simulink model "ADU_Integration_R2014a_simulation"  (R2014a)
settings: Solver=FixedStepDiscrete  StartTime=285  StopTime=300  FixedStep=0.01  RelTol=1e-3
PostLoadFcn:
  | , if any(exist('dsrtsu_mdlpostloadfcn', 'file') == [2, 3, 6]), try dsrtsu_mdlpostloadfcn('Execute', bdroot); catch fprintf('Error in PostLoadFcn (dsrtsu_mdlpostloadfcn) for model "%s":\n %s\n', bdroot, lasterr); end, end,
InitFcn:
  | load 'data/chi2_dat';
  | load 'data/Line_struct';
  | load 'data/innerLNM_1';
  | load 'data/middleLNM_2';
  | load 'data/outerLNM_1';
  | load 'data/landmarks_patac_schimmel_ccw';
  | load 'data/patac_navi_array';
  | load 'data/sensor';
  | load 'data/map_struct';
  | addpath map_src
  | Integration_Parameter;
  | load 'TestData_001';
values from neighbouring files (symbols this model uses):
  TestData_001 =     [TestData_001.mat]
undefined symbols (not defined in the file or in its folder): chi2_dat, innerLNM_1, landmarks_patac_schimmel_ccw, middleLNM_2, outerLNM_1, patac_navi_array
libraries: simulink x36, rtican x1
(part 12 of 22)

== matlab function ADU_Integration_R2014a_simulation/Path_Plan/CordTransfer ==
  data: Info_MeGCd input; Info_MePGCd output size=1,6; RoadInfoPGCd output size=2,4; Info_FdGCd input; Info_FoGCd input; Info_LdGCd input; Info_LoGCd input; CurOpGCd input; LongDisLimitGCd input; RoadInfoGCd input; Info_FdPGCd output size=1,6; Info_FoPGCd output size=1,6; Info_LdPGCd output size=1,6; Info_LoPGCd output size=1,6; LongDisLimitPGCd output; CurOpPGCd output; PGCdInfo output size=1,3
function [Info_MePGCd,RoadInfoPGCd,Info_FdPGCd,Info_FoPGCd,Info_LdPGCd,Info_LoPGCd,LongDisLimitPGCd,CurOpPGCd,PGCdInfo] = CordTransfer(Info_MeGCd,Info_FdGCd,Info_FoGCd,Info_LdGCd,Info_LoGCd,CurOpGCd,LongDisLimitGCd,RoadInfoGCd)
%#codegen
%RoadInfo(1,1) = Info_Me(1);RoadInfo(1,2) = Info_Me(2);RoadInfo(1,3) = Info_Me(6);RoadInfo(1,4) = EgoLaneInfo(2);
    persistent CurOpTemp PGCXorig PGCYorig PGCThetaorig
    if isempty(CurOpTemp)
        CurOpTemp = 0;
    end
    if isempty(PGCXorig)
        PGCXorig = 0;
    end
    if isempty(PGCYorig)
        PGCYorig = 0;
    end
    if isempty(PGCThetaorig)
        PGCThetaorig = 0;
    end
    Info_MePGCd = [0 0 0 0 0 0];Info_FdPGCd = [0 0 0 0 0 0];Info_FoPGCd = [0 0 0 0 0 0];Info_LdPGCd = [0 0 0 0 0 0];Info_LoPGCd = [0 0 0 0 0 0];LongDisLimitPGCd = 0;RoadInfoPGCd = [0 0 0 0;0 0 0 0];PGCdInfo = [0 0 0];
    LongDisLimitPGCd = LongDisLimitGCd;CurOpPGCd = CurOpGCd;
    if abs(CurOpTemp - CurOpGCd) >1e-1
        CurOpTemp = CurOpGCd;
        PGCXorig = RoadInfoGCd(1,1);
        PGCYorig = RoadInfoGCd(1,2);
        PGCThetaorig = RoadInfoGCd(1,3);
    else
    end
    Info_MePGCd = Info_MeGCd;RoadInfoPGCd = RoadInfoGCd;Info_FdPGCd = Info_FdGCd;Info_FoPGCd = Info_FoGCd;Info_LdPGCd = Info_LdGCd;Info_LoPGCd = Info_LoGCd;
    % Transform only when there is an operation
    if CurOpGCd > 1e-1
    %     theta_rot = angle_in;
        %     x_outRot = (x_out - x_in)*cos(theta_rot) + (y_out - y_in)*sin(theta_rot);
        %     y_outRot = (y_out - y_in)*cos(theta_rot) - (x_out - x_in)*sin(theta_rot);    
        % X Y Rot and Move
        Info_MePGCd(1) = (Info_MeGCd(1) - PGCXorig)*cos(PGCThetaorig) + (Info_MeGCd(2) - PGCYorig)*sin(PGCThetaorig); 
        Info_MePGCd(2) = (Info_MeGCd(2) - PGCYorig)*cos(PGCThetaorig) - (Info_MeGCd(1) - PGCXorig)*sin(PGCThetaorig); 
        Info_FdPGCd(1) = (Info_FdGCd(1) - PGCXorig)*cos(PGCThetaorig) + (Info_FdGCd(2) - PGCYorig)*sin(PGCThetaorig); 
        Info_FdPGCd(2) = (Info_FdGCd(2) - PGCYorig)*cos(PGCThetaorig) - (Info_FdGCd(1) - PGCXorig)*sin(PGCThetaorig); 
        Info_FoPGCd(1) = (Info_FoGCd(1) - PGCXorig)*cos(PGCThetaorig) + (Info_FoGCd(2) - PGCYorig)*sin(PGCThetaorig); 
        Info_FoPGCd(2) = (Info_FoGCd(2) - PGCYorig)*cos(PGCThetaorig) - (Info_FoGCd(1) - PGCXorig)*sin(PGCThetaorig); 
        Info_LdPGCd(1) = (Info_LdGCd(1) - PGCXorig)*cos(PGCThetaorig) + (Info_LdGCd(2) - PGCYorig)*sin(PGCThetaorig); 
        Info_LdPGCd(2) = (Info_LdGCd(2) - PGCYorig)*cos(PGCThetaorig) - (Info_LdGCd(1) - PGCXorig)*sin(PGCThetaorig); 
        Info_LoPGCd(1) = (Info_LoGCd(1) - PGCXorig)*cos(PGCThetaorig) + (Info_LoGCd(2) - PGCYorig)*sin(PGCThetaorig); 
        Info_LoPGCd(2) = (Info_LoGCd(2) - PGCYorig)*cos(PGCThetaorig) - (Info_LoGCd(1) - PGCXorig)*sin(PGCThetaorig); 
        RoadInfoPGCd(1,1) = (RoadInfoGCd(1,1) - PGCXorig)*cos(PGCThetaorig) + (RoadInfoGCd(1,2) - PGCYorig)*sin(PGCThetaorig); 
        RoadInfoPGCd(1,2) = (RoadInfoGCd(1,2) - PGCYorig)*cos(PGCThetaorig) - (RoadInfoGCd(1,1) - PGCXorig)*sin(PGCThetaorig);    
        RoadInfoPGCd(2,1) = (RoadInfoGCd(2,1) - PGCXorig)*cos(PGCThetaorig) + (RoadInfoGCd(2,2) - PGCYorig)*sin(PGCThetaorig); 
        RoadInfoPGCd(2,2) = (RoadInfoGCd(2,2) - PGCYorig)*cos(PGCThetaorig) - (RoadInfoGCd(2,1) - PGCXorig)*sin(PGCThetaorig); 
        %Angle Rot
        Info_MePGCd(6) = Info_MeGCd(6) - PGCThetaorig;
        Info_FdPGCd(6) = Info_FdGCd(6) - PGCThetaorig;
        Info_FoPGCd(6) = Info_FoGCd(6) - PGCThetaorig;
        Info_LdPGCd(6) = Info_LdGCd(6) - PGCThetaorig;      
        Info_LoPGCd(6) = Info_LoGCd(6) - PGCThetaorig;
        RoadInfoPGCd(1,3) = RoadInfoGCd(1,3) - PGCThetaorig;
        RoadInfoPGCd(2,3) = RoadInfoGCd(2,3) - PGCThetaorig;
        PGCdInfo = [PGCXorig,PGCYorig,PGCThetaorig];   
    else
        PGCXorig = 0;
        PGCYorig = 0;
        PGCThetaorig = 0;        
    end
 
end

== matlab function ADU_Integration_R2014a_simulation/Path_Plan/CordTransfer1 ==
  data: PGCdInfo input; VsPathPlan_h_positionPGC input; VsPathPlan_h_position output; VsPathPlan_h_MotionPGC input; TargetThetaLoPGC input; VsPathPlan_h_Motion output; TargetThetaLo output
function [VsPathPlan_h_position,VsPathPlan_h_Motion,TargetThetaLo] = CordTransfer(PGCdInfo,VsPathPlan_h_positionPGC,VsPathPlan_h_MotionPGC,TargetThetaLoPGC)
%#codegen
%RoadInfo(1,1) = Info_Me(1);RoadInfo(1,2) = Info_Me(2);RoadInfo(1,3) = Info_Me(6);RoadInfo(1,4) = EgoLaneInfo(2);
VsPathPlan_h_position = VsPathPlan_h_positionPGC;
VsPathPlan_h_Motion = VsPathPlan_h_MotionPGC;
TargetThetaLo = TargetThetaLoPGC;
end

== stateflow chart ADU_Integration_R2014a_simulation/Fusion_Model/Fusion_Block/Side_Fusion/RR_SRR_CoordinateAlig ==
  state [rangeX,rangeY] = TemporalAligRR(range,azimuth,W,L,InstallAngRRSRR) [function]
  (default) -> (junction 95) : {
      | k=0;
      | RRSRR_Output=0;
      | }
  (junction 95) -> (junction 98) [order 1] : [k<10]
  (junction 98) -> (junction 104) [order 1] : [RRSRR_Input[k][0]!=0]
  (junction 101) -> (junction 95) : {
      | k++;
      | }
  (junction 95) -> (junction 96) [order 2] : {
      | SideFusion;
      | }
  (junction 98) -> (junction 101) [order 2]
  (junction 104) -> (junction 106) : {
      | RRSRR_Output[k][0]=RRSRR_Input[k][0];%Target ID
      | [RRSRR_Output[k][1],RRSRR_Output[k][2]]=TemporalAligRR(RRSRR_Input[k][1],RRSRR_Input[k][2],W,L,InstallAng*3.1415/180);
      | RRSRR_Output[k][3]=RRSRR_Input[k][4]; %Target DynamicMode
      | }
  (junction 106) -> (junction 101)
  data: range function_input; rangeX function_output; rangeY function_output; azimuth function_input; W function_input double size=1; L function_input double size=1; InstallAngRRSRR function_input double size=1; RRSRR_Input input double size=[10 5]; RRSRR_Output output double size=[10 4]; k local double size=1 =0; L constant double =5.2; W constant double =1.8; InstallAng constant double =60
  events: SRR_Trig input EITHER_EDGE_EVENT; SideFusion output FUNCTION_CALL_EVENT

== stateflow chart ADU_Integration_R2014a_simulation/LogData/Sensor_ESR/Chart ==
  (default) -> (junction 14) : {
      | k=0;
      | TargetNum=0;
      | DataOutput=0;
      | }
  (junction 14) -> (junction 25) [order 1] : [k<64]
  (junction 25) -> (junction 30) [order 1] : [DataInput[k][3]!=0]
  (junction 28) -> (junction 14) : {
      | k++;
      | }
  (junction 14) -> (junction 16) [order 2]
  (junction 25) -> (junction 28) [order 2]
  (junction 30) -> (junction 33) : {
      | DataOutput[TargetNum][0]=DataInput[k][0];
      | DataOutput[TargetNum][1]=DataInput[k][1];
      | DataOutput[TargetNum][2]=DataInput[k][2];
      | DataOutput[TargetNum][3]=DataInput[k][3];
      | TargetNum++;
      | }
  (junction 33) -> (junction 28)
  (junction 16) -> (junction 17)
  data: DataInput input size=[64 4]; DataOutput output double size=[64 4]; k local double size=1 =0; TargetNum local double size=1 =0
  events: Trigger input EITHER_EDGE_EVENT

== stateflow chart ADU_Integration_R2014a_simulation/LogData/LF_SRR_Data/Chart ==
  (default) -> (junction 13)
  (junction 13) -> (junction 14) [order 1] : [Trig != preTrig]
  (junction 13) -> (junction 15) [order 2]
  (junction 14) -> (junction 16) : {
      | DataOutput=DataInput;
      | Time_out=Time;
      | }
  (junction 16) -> (junction 15)
  (junction 15) -> (junction 17) : {
      | preTrig=Trig;
      | }
  data: Trig input; DataInput input size=[10 5]; DataOutput output double size=[10 5]; Time input; preTrig local double; Time_out output double

== stateflow chart ADU_Integration_R2014a_simulation/LogData/Sensor_ESR/Chart2 ==
  state B
  state B1
  (default) -> B : {count=0;}
  B -> B1 : {
      | count=count+1;
      | }
  B1 -> B : {
      | count=count-1;
      | }
  data: count output double
  events: event input FUNCTION_CALL_EVENT

== stateflow chart ADU_Integration_R2014a_simulation/Fusion_Model/Fusion_Block/Side_Fusion/SRR_Data_Out ==
  (default) -> (junction 113) : {
      | k=0;
      | SRR_Data=0;
      | SideFusNum=0;
      | }
  (junction 113) -> (junction 115) [order 1] : [k<10]
  (junction 118) -> (junction 113) : {
      | k++;
      | }
  (junction 113) -> (junction 129) [order 2] : {
      | k=0;
      | }
  (junction 115) -> (junction 118) : {
      | SRR_Data[SideFusNum][0]=LFSRR_Input[k][0];SRR_Data[SideFusNum][1]=LFSRR_Input[k][1];
      | SRR_Data[SideFusNum][2]=LFSRR_Input[k][2];SRR_Data[SideFusNum][3]=LFSRR_Input[k][3];
      | SideFusNum=SideFusNum+1;
      | }
  (junction 129) -> (junction 136) [order 1] : [k<10]
  (junction 140) -> (junction 129) : {
      | k++;
      | }
  (junction 129) -> (junction 151) [order 2] : {
      | k=0;
      | }
  (junction 136) -> (junction 140) : {
      | SRR_Data[SideFusNum][0]=RFSRR_Input[k][0];SRR_Data[SideFusNum][1]=RFSRR_Input[k][1];
      | SRR_Data[SideFusNum][2]=RFSRR_Input[k][2];SRR_Data[SideFusNum][3]=RFSRR_Input[k][3];
      | SideFusNum=SideFusNum+1;
      | }
  (junction 151) -> (junction 149) [order 1] : [k<10]
  (junction 145) -> (junction 151) : {
      | k++;
      | }
  (junction 151) -> (junction 160) [order 2] : {
      | k=0;
      | }
  (junction 149) -> (junction 145) : {
      | SRR_Data[SideFusNum][0]=LRSRR_Input[k][0];SRR_Data[SideFusNum][1]=LRSRR_Input[k][1];
      | SRR_Data[SideFusNum][2]=LRSRR_Input[k][2];SRR_Data[SideFusNum][3]=LRSRR_Input[k][3];
      | SideFusNum=SideFusNum+1;
      | }
  (junction 160) -> (junction 164) [order 1] : [k<10]
  (junction 159) -> (junction 160) : {
      | k++;
      | }
  (junction 160) -> (junction 172) [order 2]
  (junction 164) -> (junction 159) : {
      | SRR_Data[SideFusNum][0]=RRSRR_Input[k][0];SRR_Data[SideFusNum][1]=RRSRR_Input[k][1];
      | SRR_Data[SideFusNum][2]=RRSRR_Input[k][2];SRR_Data[SideFusNum][3]=RRSRR_Input[k][3];
      | SideFusNum=SideFusNum+1;
      | }
  data: LFSRR_Input input double size=[10 4]; RFSRR_Input input double size=[10 4]; LRSRR_Input input double size=[10 4]; RRSRR_Input input double size=[10 4]; SRR_Data output double size=[40 4]; k local double size=1 =0; count local double size=1 =0; SideFusNum local double size=1 =0

== matlab function ADU_Integration_R2014a_simulation/Path_Plan/InterSectionPathPlanningModule/MATLAB Function ==
  data: CurOp input; TrigFlg output
function TrigFlg = OpTrigJudge(CurOp)
%#codegen
    %Operation 0 NA    %Operation 1 RT    %Operation 2 LT    %Operation 3 ST    %Operation 4 PK    %Operation 5 LC    %Operation 6 Transition
    persistent TrigEventEdge
    if isempty(TrigEventEdge)
        TrigEventEdge = 0;
    end
    TrigFlg = 0;
    if (abs(CurOp - 1)<1e-1) || ( abs(CurOp - 2)<1e-1)  
        TrigEdgeResCur = 1;
    else
        TrigEdgeResCur = 0;  
    end

    if ((abs(TrigEventEdge - TrigEdgeResCur) > 1e-1)) 
        if (TrigEdgeResCur > 1e-1)
            TrigFlg = 1;
        else
        end
        TrigEventEdge = TrigEdgeResCur;
    else
        TrigFlg = 0;
    end 
end

== stateflow chart ADU_Integration_R2014a_simulation/LogData/RF_SRR_Data/Chart ==
  (default) -> (junction 13)
  (junction 13) -> (junction 14) [order 1] : [Trig != preTrig]
  (junction 13) -> (junction 15) [order 2]
  (junction 14) -> (junction 16) : {
      | DataOutput=DataInput;
      | Time_out=Time;
      | }
  (junction 16) -> (junction 15)
  (junction 15) -> (junction 17) : {
      | preTrig=Trig;
      | }
  data: Trig input; DataInput input size=[10 5]; DataOutput output double size=[10 5]; Time input; preTrig local double; Time_out output double

== matlab function ADU_Integration_R2014a_simulation/Path_Plan/InterSectionPathPlanningModule/MATLAB Function1 ==
  data: RoadInfo input; x_in output; y_in output; angle_in output; x_out output; y_out output; angle_out output; W_in output; W_out output
function [x_in,y_in,angle_in,x_out,y_out,angle_out,W_in,W_out] = RoadInfoDistribute(RoadInfo)
%#codegen
%         RoadInfo(1,1) = Info_Me(1);RoadInfo(1,2) = Info_Me(2);RoadInfo(1,3) = Info_Me(6);RoadInfo(1,4) = EgoLaneInfo(2);
%         RoadInfo(2,:) = [EgoLaneInfo(3),EgoLaneInfo(4),EgoLaneInfo(1),EgoLaneInfo(2)]; 
    x_in = RoadInfo(1,1);y_in = RoadInfo(1,2);angle_in = RoadInfo(1,3);W_in = RoadInfo(1,4);
    x_out = RoadInfo(2,1);y_out = RoadInfo(2,2);angle_out = RoadInfo(2,3); W_out = RoadInfo(2,4);
end

== stateflow chart ADU_Integration_R2014a_simulation/LogData/LR_SRR_Data/Chart ==
  (default) -> (junction 13)
  (junction 13) -> (junction 14) [order 1] : [Trig != preTrig]
  (junction 13) -> (junction 15) [order 2]
  (junction 14) -> (junction 16) : {
      | DataOutput=DataInput;
      | Time_out=Time;
      | }
  (junction 16) -> (junction 15)
  (junction 15) -> (junction 17) : {
      | preTrig=Trig;
      | }
  data: Trig input; DataInput input size=[10 5]; DataOutput output double size=[10 5]; Time input; preTrig local double; Time_out output double
